simulink model "ZeroForceDrag_SingleJoint"  (R2018b)
settings: Solver=FixedStepDiscrete  StartTime=0.0  StopTime=Inf  FixedStep=0.001  RelTol=1e-3  EnableMultiTasking=on
undefined symbols (not defined in the file): J1, J2, J3, J4, J5, J6, J7, Motor_Current, Motor_Position, Motor_Velocity, Send_GUIdata
libraries: c280xlib x14, simulink x5, idelinklib_common x1
(part 3 of 4)

== system ZeroForceDrag_SingleJoint/DynamicCalculation/GetAngleVelocity/GetAngle2/Joint5 ==
  Action Port : ActionPort  ActionType=case
  Data Store Read5 : DataStoreRead  DataStoreName=Motor_Position  DataStoreElements=Motor_Position(5)
  Joint5 : Outport
  wires:
  Data Store Read5/1 -> Joint5/1

== system ZeroForceDrag_SingleJoint/DynamicCalculation/GetAngleVelocity/GetAngle2/Joint6 ==
  Action Port : ActionPort  ActionType=case
  Data Store Read5 : DataStoreRead  DataStoreName=Motor_Position  DataStoreElements=Motor_Position(6)
  Joint6 : Outport
  wires:
  Data Store Read5/1 -> Joint6/1

== system ZeroForceDrag_SingleJoint/DynamicCalculation/GetAngleVelocity/GetAngle3/Joint1 ==
  note: 内转子位置的脉冲值
  Action Port : ActionPort  ActionType=case
  Data Store Read5 : DataStoreRead  DataStoreName=Motor_Position  DataStoreElements=Motor_Position(1)
  Joint1 : Outport
  wires:
  Data Store Read5/1 -> Joint1/1

== system ZeroForceDrag_SingleJoint/DynamicCalculation/GetAngleVelocity/GetAngle3/Joint2 ==
  Action Port : ActionPort  ActionType=case
  Data Store Read5 : DataStoreRead  DataStoreName=Motor_Position  DataStoreElements=Motor_Position(2)
  Joint2 : Outport
  wires:
  Data Store Read5/1 -> Joint2/1

== system ZeroForceDrag_SingleJoint/DynamicCalculation/GetAngleVelocity/GetAngle3/Joint3 ==
  Action Port : ActionPort  ActionType=case
  Data Store Read5 : DataStoreRead  DataStoreName=Motor_Position  DataStoreElements=Motor_Position(3)
  Joint3 : Outport
  wires:
  Data Store Read5/1 -> Joint3/1

== system ZeroForceDrag_SingleJoint/DynamicCalculation/GetAngleVelocity/GetAngle3/Joint4 ==
  Action Port : ActionPort  ActionType=case
  Data Store Read5 : DataStoreRead  DataStoreName=Motor_Position  DataStoreElements=Motor_Position(4)
  Joint4 : Outport
  wires:
  Data Store Read5/1 -> Joint4/1

== system ZeroForceDrag_SingleJoint/DynamicCalculation/GetAngleVelocity/GetAngle3/Joint5 ==
  Action Port : ActionPort  ActionType=case
  Data Store Read5 : DataStoreRead  DataStoreName=Motor_Position  DataStoreElements=Motor_Position(5)
  Joint5 : Outport
  wires:
  Data Store Read5/1 -> Joint5/1

== system ZeroForceDrag_SingleJoint/DynamicCalculation/GetAngleVelocity/GetAngle3/Joint6 ==
  Action Port : ActionPort  ActionType=case
  Data Store Read5 : DataStoreRead  DataStoreName=Motor_Position  DataStoreElements=Motor_Position(6)
  Joint6 : Outport
  wires:
  Data Store Read5/1 -> Joint6/1

== system ZeroForceDrag_SingleJoint/DynamicCalculation/GetAngleVelocity/GetAngle4/Joint1 ==
  note: 内转子位置的脉冲值
  Action Port : ActionPort  ActionType=case
  Data Store Read5 : DataStoreRead  DataStoreName=Motor_Position  DataStoreElements=Motor_Position(1)
  Joint1 : Outport
  wires:
  Data Store Read5/1 -> Joint1/1

== system ZeroForceDrag_SingleJoint/DynamicCalculation/GetAngleVelocity/GetAngle4/Joint2 ==
  Action Port : ActionPort  ActionType=case
  Data Store Read5 : DataStoreRead  DataStoreName=Motor_Position  DataStoreElements=Motor_Position(2)
  Joint2 : Outport
  wires:
  Data Store Read5/1 -> Joint2/1

== system ZeroForceDrag_SingleJoint/DynamicCalculation/GetAngleVelocity/GetAngle4/Joint3 ==
  Action Port : ActionPort  ActionType=case
  Data Store Read5 : DataStoreRead  DataStoreName=Motor_Position  DataStoreElements=Motor_Position(3)
  Joint3 : Outport
  wires:
  Data Store Read5/1 -> Joint3/1

== system ZeroForceDrag_SingleJoint/DynamicCalculation/GetAngleVelocity/GetAngle4/Joint4 ==
  Action Port : ActionPort  ActionType=case
  Data Store Read5 : DataStoreRead  DataStoreName=Motor_Position  DataStoreElements=Motor_Position(4)
  Joint4 : Outport
  wires:
  Data Store Read5/1 -> Joint4/1

== system ZeroForceDrag_SingleJoint/DynamicCalculation/GetAngleVelocity/GetAngle4/Joint5 ==
  Action Port : ActionPort  ActionType=case
  Data Store Read5 : DataStoreRead  DataStoreName=Motor_Position  DataStoreElements=Motor_Position(5)
  Joint5 : Outport
  wires:
  Data Store Read5/1 -> Joint5/1

== system ZeroForceDrag_SingleJoint/DynamicCalculation/GetAngleVelocity/GetAngle4/Joint6 ==
  Action Port : ActionPort  ActionType=case
  Data Store Read5 : DataStoreRead  DataStoreName=Motor_Position  DataStoreElements=Motor_Position(6)
  Joint6 : Outport
  wires:
  Data Store Read5/1 -> Joint6/1

== system ZeroForceDrag_SingleJoint/DynamicCalculation/GetAngleVelocity/GetAngle5/Joint1 ==
  note: 内转子位置的脉冲值
  Action Port : ActionPort  ActionType=case
  Data Store Read5 : DataStoreRead  DataStoreName=Motor_Position  DataStoreElements=Motor_Position(1)
  Joint1 : Outport
  wires:
  Data Store Read5/1 -> Joint1/1

== system ZeroForceDrag_SingleJoint/DynamicCalculation/GetAngleVelocity/GetAngle5/Joint2 ==
  Action Port : ActionPort  ActionType=case
  Data Store Read5 : DataStoreRead  DataStoreName=Motor_Position  DataStoreElements=Motor_Position(2)
  Joint2 : Outport
  wires:
  Data Store Read5/1 -> Joint2/1

== system ZeroForceDrag_SingleJoint/DynamicCalculation/GetAngleVelocity/GetAngle5/Joint3 ==
  Action Port : ActionPort  ActionType=case
  Data Store Read5 : DataStoreRead  DataStoreName=Motor_Position  DataStoreElements=Motor_Position(3)
  Joint3 : Outport
  wires:
  Data Store Read5/1 -> Joint3/1

== system ZeroForceDrag_SingleJoint/DynamicCalculation/GetAngleVelocity/GetAngle5/Joint4 ==
  Action Port : ActionPort  ActionType=case
  Data Store Read5 : DataStoreRead  DataStoreName=Motor_Position  DataStoreElements=Motor_Position(4)
  Joint4 : Outport
  wires:
  Data Store Read5/1 -> Joint4/1

== system ZeroForceDrag_SingleJoint/DynamicCalculation/GetAngleVelocity/GetAngle5/Joint5 ==
  Action Port : ActionPort  ActionType=case
  Data Store Read5 : DataStoreRead  DataStoreName=Motor_Position  DataStoreElements=Motor_Position(5)
  Joint5 : Outport
  wires:
  Data Store Read5/1 -> Joint5/1

== system ZeroForceDrag_SingleJoint/DynamicCalculation/GetAngleVelocity/GetAngle5/Joint6 ==
  Action Port : ActionPort  ActionType=case
  Data Store Read5 : DataStoreRead  DataStoreName=Motor_Position  DataStoreElements=Motor_Position(6)
  Joint6 : Outport
  wires:
  Data Store Read5/1 -> Joint6/1

== system ZeroForceDrag_SingleJoint/DynamicCalculation/GetAngleVelocity/GetAngle6/Joint1 ==
  note: 内转子位置的脉冲值
  Action Port : ActionPort  ActionType=case
  Data Store Read5 : DataStoreRead  DataStoreName=Motor_Position  DataStoreElements=Motor_Position(1)
  Joint1 : Outport
  wires:
  Data Store Read5/1 -> Joint1/1

== system ZeroForceDrag_SingleJoint/DynamicCalculation/GetAngleVelocity/GetAngle6/Joint2 ==
  Action Port : ActionPort  ActionType=case
  Data Store Read5 : DataStoreRead  DataStoreName=Motor_Position  DataStoreElements=Motor_Position(2)
  Joint2 : Outport
  wires:
  Data Store Read5/1 -> Joint2/1

== system ZeroForceDrag_SingleJoint/DynamicCalculation/GetAngleVelocity/GetAngle6/Joint3 ==
  Action Port : ActionPort  ActionType=case
  Data Store Read5 : DataStoreRead  DataStoreName=Motor_Position  DataStoreElements=Motor_Position(3)
  Joint3 : Outport
  wires:
  Data Store Read5/1 -> Joint3/1

== system ZeroForceDrag_SingleJoint/DynamicCalculation/GetAngleVelocity/GetAngle6/Joint4 ==
  Action Port : ActionPort  ActionType=case
  Data Store Read5 : DataStoreRead  DataStoreName=Motor_Position  DataStoreElements=Motor_Position(4)
  Joint4 : Outport
  wires:
  Data Store Read5/1 -> Joint4/1

== system ZeroForceDrag_SingleJoint/DynamicCalculation/GetAngleVelocity/GetAngle6/Joint5 ==
  Action Port : ActionPort  ActionType=case
  Data Store Read5 : DataStoreRead  DataStoreName=Motor_Position  DataStoreElements=Motor_Position(5)
  Joint5 : Outport
  wires:
  Data Store Read5/1 -> Joint5/1

== system ZeroForceDrag_SingleJoint/DynamicCalculation/GetAngleVelocity/GetAngle6/Joint6 ==
  Action Port : ActionPort  ActionType=case
  Data Store Read5 : DataStoreRead  DataStoreName=Motor_Position  DataStoreElements=Motor_Position(6)
  Joint6 : Outport
  wires:
  Data Store Read5/1 -> Joint6/1

== system ZeroForceDrag_SingleJoint/DynamicCalculation/GetAngleVelocity/GetAngleSpeed/Joint1 ==
  note: 内转子速度
      | 的脉冲值
  Action Port : ActionPort  ActionType=case
  Data Store Read1 : DataStoreRead  DataStoreName=Motor_Velocity  DataStoreElements=Motor_Velocity(1)
  Joint1_Velocity : Outport
  wires:
  Data Store Read1/1 -> Joint1_Velocity/1

== system ZeroForceDrag_SingleJoint/DynamicCalculation/GetAngleVelocity/GetAngleSpeed/Joint2 ==
  note: 内转子速度
      | 的脉冲值
  Action Port : ActionPort  ActionType=case
  Data Store Read1 : DataStoreRead  DataStoreName=Motor_Velocity  DataStoreElements=Motor_Velocity(2)
  Joint2_Velocity : Outport
  wires:
  Data Store Read1/1 -> Joint2_Velocity/1

== system ZeroForceDrag_SingleJoint/DynamicCalculation/GetAngleVelocity/GetAngleSpeed/Joint3 ==
  note: 内转子速度
      | 的脉冲值
  Action Port : ActionPort  ActionType=case
  Data Store Read1 : DataStoreRead  DataStoreName=Motor_Velocity  DataStoreElements=Motor_Velocity(3)
  Joint3_Velocity : Outport
  wires:
  Data Store Read1/1 -> Joint3_Velocity/1

== system ZeroForceDrag_SingleJoint/DynamicCalculation/GetAngleVelocity/GetAngleSpeed/Joint4 ==
  note: 内转子速度
      | 的脉冲值
  Action Port : ActionPort  ActionType=case
  Data Store Read1 : DataStoreRead  DataStoreName=Motor_Velocity  DataStoreElements=Motor_Velocity(4)
  Joint4_Velocity : Outport
  wires:
  Data Store Read1/1 -> Joint4_Velocity/1

== system ZeroForceDrag_SingleJoint/DynamicCalculation/GetAngleVelocity/GetAngleSpeed/Joint5 ==
  note: 内转子速度
      | 的脉冲值
  Action Port : ActionPort  ActionType=case
  Data Store Read1 : DataStoreRead  DataStoreName=Motor_Velocity  DataStoreElements=Motor_Velocity(5)
  Joint5_Velocity : Outport
  wires:
  Data Store Read1/1 -> Joint5_Velocity/1

== system ZeroForceDrag_SingleJoint/DynamicCalculation/GetAngleVelocity/GetAngleSpeed/Joint6 ==
  note: 内转子速度
      | 的脉冲值
  Action Port : ActionPort  ActionType=case
  Data Store Read1 : DataStoreRead  DataStoreName=Motor_Velocity  DataStoreElements=Motor_Velocity(6)
  Joint6_Velocity : Outport
  wires:
  Data Store Read1/1 -> Joint6_Velocity/1

== system ZeroForceDrag_SingleJoint/DynamicCalculation/GetAngleVelocity/GetAngleSpeed1/Joint1 ==
  note: 内转子速度
      | 的脉冲值
  Action Port : ActionPort  ActionType=case
  Data Store Read1 : DataStoreRead  DataStoreName=Motor_Velocity  DataStoreElements=Motor_Velocity(1)
  Joint1_Velocity : Outport
  wires:
  Data Store Read1/1 -> Joint1_Velocity/1

== system ZeroForceDrag_SingleJoint/DynamicCalculation/GetAngleVelocity/GetAngleSpeed1/Joint2 ==
  note: 内转子速度
      | 的脉冲值
  Action Port : ActionPort  ActionType=case
  Data Store Read1 : DataStoreRead  DataStoreName=Motor_Velocity  DataStoreElements=Motor_Velocity(2)
  Joint2_Velocity : Outport
  wires:
  Data Store Read1/1 -> Joint2_Velocity/1

== system ZeroForceDrag_SingleJoint/DynamicCalculation/GetAngleVelocity/GetAngleSpeed1/Joint3 ==
  note: 内转子速度
      | 的脉冲值
  Action Port : ActionPort  ActionType=case
  Data Store Read1 : DataStoreRead  DataStoreName=Motor_Velocity  DataStoreElements=Motor_Velocity(3)
  Joint3_Velocity : Outport
  wires:
  Data Store Read1/1 -> Joint3_Velocity/1

== system ZeroForceDrag_SingleJoint/DynamicCalculation/GetAngleVelocity/GetAngleSpeed1/Joint4 ==
  note: 内转子速度
      | 的脉冲值
  Action Port : ActionPort  ActionType=case
  Data Store Read1 : DataStoreRead  DataStoreName=Motor_Velocity  DataStoreElements=Motor_Velocity(4)
  Joint4_Velocity : Outport
  wires:
  Data Store Read1/1 -> Joint4_Velocity/1

== system ZeroForceDrag_SingleJoint/DynamicCalculation/GetAngleVelocity/GetAngleSpeed1/Joint5 ==
  note: 内转子速度
      | 的脉冲值
  Action Port : ActionPort  ActionType=case
  Data Store Read1 : DataStoreRead  DataStoreName=Motor_Velocity  DataStoreElements=Motor_Velocity(5)
  Joint5_Velocity : Outport
  wires:
  Data Store Read1/1 -> Joint5_Velocity/1

== system ZeroForceDrag_SingleJoint/DynamicCalculation/GetAngleVelocity/GetAngleSpeed1/Joint6 ==
  note: 内转子速度
      | 的脉冲值
  Action Port : ActionPort  ActionType=case
  Data Store Read1 : DataStoreRead  DataStoreName=Motor_Velocity  DataStoreElements=Motor_Velocity(6)
  Joint6_Velocity : Outport
  wires:
  Data Store Read1/1 -> Joint6_Velocity/1

== system ZeroForceDrag_SingleJoint/DynamicCalculation/GetAngleVelocity/GetAngleSpeed2/Joint1 ==
  note: 内转子速度
      | 的脉冲值
  Action Port : ActionPort  ActionType=case
  Data Store Read1 : DataStoreRead  DataStoreName=Motor_Velocity  DataStoreElements=Motor_Velocity(1)
  Joint1_Velocity : Outport
  wires:
  Data Store Read1/1 -> Joint1_Velocity/1

== system ZeroForceDrag_SingleJoint/DynamicCalculation/GetAngleVelocity/GetAngleSpeed2/Joint2 ==
  note: 内转子速度
      | 的脉冲值
  Action Port : ActionPort  ActionType=case
  Data Store Read1 : DataStoreRead  DataStoreName=Motor_Velocity  DataStoreElements=Motor_Velocity(2)
  Joint2_Velocity : Outport
  wires:
  Data Store Read1/1 -> Joint2_Velocity/1

== system ZeroForceDrag_SingleJoint/DynamicCalculation/GetAngleVelocity/GetAngleSpeed2/Joint3 ==
  note: 内转子速度
      | 的脉冲值
  Action Port : ActionPort  ActionType=case
  Data Store Read1 : DataStoreRead  DataStoreName=Motor_Velocity  DataStoreElements=Motor_Velocity(3)
  Joint3_Velocity : Outport
  wires:
  Data Store Read1/1 -> Joint3_Velocity/1

== system ZeroForceDrag_SingleJoint/DynamicCalculation/GetAngleVelocity/GetAngleSpeed2/Joint4 ==
  note: 内转子速度
      | 的脉冲值
  Action Port : ActionPort  ActionType=case
  Data Store Read1 : DataStoreRead  DataStoreName=Motor_Velocity  DataStoreElements=Motor_Velocity(4)
  Joint4_Velocity : Outport
  wires:
  Data Store Read1/1 -> Joint4_Velocity/1

== system ZeroForceDrag_SingleJoint/DynamicCalculation/GetAngleVelocity/GetAngleSpeed2/Joint5 ==
  note: 内转子速度
      | 的脉冲值
  Action Port : ActionPort  ActionType=case
  Data Store Read1 : DataStoreRead  DataStoreName=Motor_Velocity  DataStoreElements=Motor_Velocity(5)
  Joint5_Velocity : Outport
  wires:
  Data Store Read1/1 -> Joint5_Velocity/1

== system ZeroForceDrag_SingleJoint/DynamicCalculation/GetAngleVelocity/GetAngleSpeed2/Joint6 ==
  note: 内转子速度
      | 的脉冲值
  Action Port : ActionPort  ActionType=case
  Data Store Read1 : DataStoreRead  DataStoreName=Motor_Velocity  DataStoreElements=Motor_Velocity(6)
  Joint6_Velocity : Outport
  wires:
  Data Store Read1/1 -> Joint6_Velocity/1

== system ZeroForceDrag_SingleJoint/DynamicCalculation/GetAngleVelocity/GetAngleSpeed3/Joint1 ==
  note: 内转子速度
      | 的脉冲值
  Action Port : ActionPort  ActionType=case
  Data Store Read1 : DataStoreRead  DataStoreName=Motor_Velocity  DataStoreElements=Motor_Velocity(1)
  Joint1_Velocity : Outport
  wires:
  Data Store Read1/1 -> Joint1_Velocity/1

== system ZeroForceDrag_SingleJoint/DynamicCalculation/GetAngleVelocity/GetAngleSpeed3/Joint2 ==
  note: 内转子速度
      | 的脉冲值
  Action Port : ActionPort  ActionType=case
  Data Store Read1 : DataStoreRead  DataStoreName=Motor_Velocity  DataStoreElements=Motor_Velocity(2)
  Joint2_Velocity : Outport
  wires:
  Data Store Read1/1 -> Joint2_Velocity/1

== system ZeroForceDrag_SingleJoint/DynamicCalculation/GetAngleVelocity/GetAngleSpeed3/Joint3 ==
  note: 内转子速度
      | 的脉冲值
  Action Port : ActionPort  ActionType=case
  Data Store Read1 : DataStoreRead  DataStoreName=Motor_Velocity  DataStoreElements=Motor_Velocity(3)
  Joint3_Velocity : Outport
  wires:
  Data Store Read1/1 -> Joint3_Velocity/1

== system ZeroForceDrag_SingleJoint/DynamicCalculation/GetAngleVelocity/GetAngleSpeed3/Joint4 ==
  note: 内转子速度
      | 的脉冲值
  Action Port : ActionPort  ActionType=case
  Data Store Read1 : DataStoreRead  DataStoreName=Motor_Velocity  DataStoreElements=Motor_Velocity(4)
  Joint4_Velocity : Outport
  wires:
  Data Store Read1/1 -> Joint4_Velocity/1

== system ZeroForceDrag_SingleJoint/DynamicCalculation/GetAngleVelocity/GetAngleSpeed3/Joint5 ==
  note: 内转子速度
      | 的脉冲值
  Action Port : ActionPort  ActionType=case
  Data Store Read1 : DataStoreRead  DataStoreName=Motor_Velocity  DataStoreElements=Motor_Velocity(5)
  Joint5_Velocity : Outport
  wires:
  Data Store Read1/1 -> Joint5_Velocity/1

== system ZeroForceDrag_SingleJoint/DynamicCalculation/GetAngleVelocity/GetAngleSpeed3/Joint6 ==
  note: 内转子速度
      | 的脉冲值
  Action Port : ActionPort  ActionType=case
  Data Store Read1 : DataStoreRead  DataStoreName=Motor_Velocity  DataStoreElements=Motor_Velocity(6)
  Joint6_Velocity : Outport
  wires:
  Data Store Read1/1 -> Joint6_Velocity/1

== system ZeroForceDrag_SingleJoint/DynamicCalculation/GetAngleVelocity/GetAngleSpeed4/Joint1 ==
  note: 内转子速度
      | 的脉冲值
  Action Port : ActionPort  ActionType=case
  Data Store Read1 : DataStoreRead  DataStoreName=Motor_Velocity  DataStoreElements=Motor_Velocity(1)
  Joint1_Velocity : Outport
  wires:
  Data Store Read1/1 -> Joint1_Velocity/1

== system ZeroForceDrag_SingleJoint/DynamicCalculation/GetAngleVelocity/GetAngleSpeed4/Joint2 ==
  note: 内转子速度
      | 的脉冲值
  Action Port : ActionPort  ActionType=case
  Data Store Read1 : DataStoreRead  DataStoreName=Motor_Velocity  DataStoreElements=Motor_Velocity(2)
  Joint2_Velocity : Outport
  wires:
  Data Store Read1/1 -> Joint2_Velocity/1

== system ZeroForceDrag_SingleJoint/DynamicCalculation/GetAngleVelocity/GetAngleSpeed4/Joint3 ==
  note: 内转子速度
      | 的脉冲值
  Action Port : ActionPort  ActionType=case
  Data Store Read1 : DataStoreRead  DataStoreName=Motor_Velocity  DataStoreElements=Motor_Velocity(3)
  Joint3_Velocity : Outport
  wires:
  Data Store Read1/1 -> Joint3_Velocity/1

== system ZeroForceDrag_SingleJoint/DynamicCalculation/GetAngleVelocity/GetAngleSpeed4/Joint4 ==
  note: 内转子速度
      | 的脉冲值
  Action Port : ActionPort  ActionType=case
  Data Store Read1 : DataStoreRead  DataStoreName=Motor_Velocity  DataStoreElements=Motor_Velocity(4)
  Joint4_Velocity : Outport
  wires:
  Data Store Read1/1 -> Joint4_Velocity/1

== system ZeroForceDrag_SingleJoint/DynamicCalculation/GetAngleVelocity/GetAngleSpeed4/Joint5 ==
  note: 内转子速度
      | 的脉冲值
  Action Port : ActionPort  ActionType=case
  Data Store Read1 : DataStoreRead  DataStoreName=Motor_Velocity  DataStoreElements=Motor_Velocity(5)
  Joint5_Velocity : Outport
  wires:
  Data Store Read1/1 -> Joint5_Velocity/1

== system ZeroForceDrag_SingleJoint/DynamicCalculation/GetAngleVelocity/GetAngleSpeed4/Joint6 ==
  note: 内转子速度
      | 的脉冲值
  Action Port : ActionPort  ActionType=case
  Data Store Read1 : DataStoreRead  DataStoreName=Motor_Velocity  DataStoreElements=Motor_Velocity(6)
  Joint6_Velocity : Outport
  wires:
  Data Store Read1/1 -> Joint6_Velocity/1

== system ZeroForceDrag_SingleJoint/DynamicCalculation/GetAngleVelocity/GetAngleSpeed5/Joint1 ==
  note: 内转子速度
      | 的脉冲值
  Action Port : ActionPort  ActionType=case
  Data Store Read1 : DataStoreRead  DataStoreName=Motor_Velocity  DataStoreElements=Motor_Velocity(1)
  Joint1_Velocity : Outport
  wires:
  Data Store Read1/1 -> Joint1_Velocity/1

== system ZeroForceDrag_SingleJoint/DynamicCalculation/GetAngleVelocity/GetAngleSpeed5/Joint2 ==
  note: 内转子速度
      | 的脉冲值
  Action Port : ActionPort  ActionType=case
  Data Store Read1 : DataStoreRead  DataStoreName=Motor_Velocity  DataStoreElements=Motor_Velocity(2)
  Joint2_Velocity : Outport
  wires:
  Data Store Read1/1 -> Joint2_Velocity/1

== system ZeroForceDrag_SingleJoint/DynamicCalculation/GetAngleVelocity/GetAngleSpeed5/Joint3 ==
  note: 内转子速度
      | 的脉冲值
  Action Port : ActionPort  ActionType=case
  Data Store Read1 : DataStoreRead  DataStoreName=Motor_Velocity  DataStoreElements=Motor_Velocity(3)
  Joint3_Velocity : Outport
  wires:
  Data Store Read1/1 -> Joint3_Velocity/1

== system ZeroForceDrag_SingleJoint/DynamicCalculation/GetAngleVelocity/GetAngleSpeed5/Joint4 ==
  note: 内转子速度
      | 的脉冲值
  Action Port : ActionPort  ActionType=case
  Data Store Read1 : DataStoreRead  DataStoreName=Motor_Velocity  DataStoreElements=Motor_Velocity(4)
  Joint4_Velocity : Outport
  wires:
  Data Store Read1/1 -> Joint4_Velocity/1

== system ZeroForceDrag_SingleJoint/DynamicCalculation/GetAngleVelocity/GetAngleSpeed5/Joint5 ==
  note: 内转子速度
      | 的脉冲值
  Action Port : ActionPort  ActionType=case
  Data Store Read1 : DataStoreRead  DataStoreName=Motor_Velocity  DataStoreElements=Motor_Velocity(5)
  Joint5_Velocity : Outport
  wires:
  Data Store Read1/1 -> Joint5_Velocity/1

== system ZeroForceDrag_SingleJoint/DynamicCalculation/GetAngleVelocity/GetAngleSpeed5/Joint6 ==
  note: 内转子速度
      | 的脉冲值
  Action Port : ActionPort  ActionType=case
  Data Store Read1 : DataStoreRead  DataStoreName=Motor_Velocity  DataStoreElements=Motor_Velocity(6)
  Joint6_Velocity : Outport
  wires:
  Data Store Read1/1 -> Joint6_Velocity/1

== system ZeroForceDrag_SingleJoint/DynamicCalculation/DriveMotor/驱动器指令/Chart2/BG/J1_BG ==
  note: 命令
  note: 电流
  note: 位
      | 置
  Constant1 : Constant  Value=hex2dec('47')  OutDataTypeStr=uint8
  Constant2 : Constant  Value=0  VectorParams1D=off  OutDataTypeStr=uint8  SampleTime=-1
  Constant3 : Constant  Value=0  VectorParams1D=off  OutDataTypeStr=uint8  SampleTime=-1
  Constant8 : Constant  Value=hex2dec('42')  OutDataTypeStr=uint8
  Data Type Conversion : DataTypeConversion  OutDataTypeStr=uint16
  Data Type Conversion{1..6} (6 alike) : DataTypeConversion  OutDataTypeStr=uint8
  Mux3 : Mux  Inputs=8
  Shift Arithmetic1 : ArithShift  BitShiftNumber=8  BitShiftDirection=Right
  Shift Arithmetic2 : ArithShift  BitShiftNumber=16  BitShiftDirection=Right
  Shift Arithmetic3 : ArithShift  BitShiftNumber=24  BitShiftDirection=Right
  Shift Arithmetic4 : ArithShift  BitShiftNumber=8  BitShiftDirection=Right
  MSG : Outport
  wires:
  Shift Arithmetic2/1 -> Data Type Conversion4/1
  Shift Arithmetic4/1 -> Data Type Conversion6/1
  Constant2/1 -> Shift Arithmetic4/1, Data Type Conversion1/1
  Data Type Conversion1/1 -> Mux3/3
  Data Type Conversion3/1 -> Mux3/6
  Constant3/1 -> Data Type Conversion2/1, Shift Arithmetic1/1, Shift Arithmetic2/1, Shift Arithmetic3/1
  Data Type Conversion6/1 -> Mux3/4
  Shift Arithmetic3/1 -> Data Type Conversion5/1
  Shift Arithmetic1/1 -> Data Type Conversion3/1
  Mux3/1 -> Data Type Conversion/1
  Data Type Conversion2/1 -> Mux3/5
  Constant8/1 -> Mux3/1
  Data Type Conversion4/1 -> Mux3/7
  Data Type Conversion5/1 -> Mux3/8
  Constant1/1 -> Mux3/2
  Data Type Conversion/1 -> MSG/1

== system ZeroForceDrag_SingleJoint/DynamicCalculation/DriveMotor/驱动器指令/Chart2/BG/J2_BG ==
  note: 位
      | 置
  note: 电流
  note: 命令
  Constant1 : Constant  Value=hex2dec('47')  OutDataTypeStr=uint8
  Constant2 : Constant  Value=0  VectorParams1D=off  OutDataTypeStr=uint8  SampleTime=-1
  Constant3 : Constant  Value=0  VectorParams1D=off  OutDataTypeStr=uint8  SampleTime=-1
  Constant8 : Constant  Value=hex2dec('42')  OutDataTypeStr=uint8
  Data Type Conversion : DataTypeConversion  OutDataTypeStr=uint16
  Data Type Conversion{1..6} (6 alike) : DataTypeConversion  OutDataTypeStr=uint8
  Mux3 : Mux  Inputs=8
  Shift Arithmetic1 : ArithShift  BitShiftNumber=8  BitShiftDirection=Right
  Shift Arithmetic2 : ArithShift  BitShiftNumber=16  BitShiftDirection=Right
  Shift Arithmetic3 : ArithShift  BitShiftNumber=24  BitShiftDirection=Right
  Shift Arithmetic4 : ArithShift  BitShiftNumber=8  BitShiftDirection=Right
  MSG : Outport
  wires:
  Data Type Conversion/1 -> MSG/1
  Constant1/1 -> Mux3/2
  Data Type Conversion5/1 -> Mux3/8
  Data Type Conversion4/1 -> Mux3/7
  Constant8/1 -> Mux3/1
  Data Type Conversion2/1 -> Mux3/5
  Mux3/1 -> Data Type Conversion/1
  Shift Arithmetic1/1 -> Data Type Conversion3/1
  Shift Arithmetic3/1 -> Data Type Conversion5/1
  Data Type Conversion6/1 -> Mux3/4
  Constant3/1 -> Shift Arithmetic3/1, Shift Arithmetic2/1, Shift Arithmetic1/1, Data Type Conversion2/1
  Data Type Conversion3/1 -> Mux3/6
  Data Type Conversion1/1 -> Mux3/3
  Constant2/1 -> Data Type Conversion1/1, Shift Arithmetic4/1
  Shift Arithmetic4/1 -> Data Type Conversion6/1
  Shift Arithmetic2/1 -> Data Type Conversion4/1

== system ZeroForceDrag_SingleJoint/DynamicCalculation/DriveMotor/驱动器指令/Chart2/BG/J3_BG ==
  note: 命令
  note: 电流
  note: 位
      | 置
  Constant1 : Constant  Value=hex2dec('47')  OutDataTypeStr=uint8
  Constant2 : Constant  Value=0  VectorParams1D=off  OutDataTypeStr=uint8  SampleTime=-1
  Constant3 : Constant  Value=0  VectorParams1D=off  OutDataTypeStr=uint8  SampleTime=-1
  Constant8 : Constant  Value=hex2dec('42')  OutDataTypeStr=uint8
  Data Type Conversion : DataTypeConversion  OutDataTypeStr=uint16
  Data Type Conversion{1..6} (6 alike) : DataTypeConversion  OutDataTypeStr=uint8
  Mux3 : Mux  Inputs=8
  Shift Arithmetic1 : ArithShift  BitShiftNumber=8  BitShiftDirection=Right
  Shift Arithmetic2 : ArithShift  BitShiftNumber=16  BitShiftDirection=Right
  Shift Arithmetic3 : ArithShift  BitShiftNumber=24  BitShiftDirection=Right
  Shift Arithmetic4 : ArithShift  BitShiftNumber=8  BitShiftDirection=Right
  MSG : Outport
  wires:
  Shift Arithmetic2/1 -> Data Type Conversion4/1
  Shift Arithmetic4/1 -> Data Type Conversion6/1
  Constant2/1 -> Shift Arithmetic4/1, Data Type Conversion1/1
  Data Type Conversion1/1 -> Mux3/3
  Data Type Conversion3/1 -> Mux3/6
  Constant3/1 -> Data Type Conversion2/1, Shift Arithmetic1/1, Shift Arithmetic2/1, Shift Arithmetic3/1
  Data Type Conversion6/1 -> Mux3/4
  Shift Arithmetic3/1 -> Data Type Conversion5/1
  Shift Arithmetic1/1 -> Data Type Conversion3/1
  Mux3/1 -> Data Type Conversion/1
  Data Type Conversion2/1 -> Mux3/5
  Constant8/1 -> Mux3/1
  Data Type Conversion4/1 -> Mux3/7
  Data Type Conversion5/1 -> Mux3/8
  Constant1/1 -> Mux3/2
  Data Type Conversion/1 -> MSG/1

== system ZeroForceDrag_SingleJoint/DynamicCalculation/DriveMotor/驱动器指令/Chart2/BG/J4_BG ==
  note: 位
      | 置
  note: 电流
  note: 命令
  Constant1 : Constant  Value=hex2dec('47')  OutDataTypeStr=uint8
  Constant2 : Constant  Value=0  VectorParams1D=off  OutDataTypeStr=uint8  SampleTime=-1
  Constant3 : Constant  Value=0  VectorParams1D=off  OutDataTypeStr=uint8  SampleTime=-1
  Constant8 : Constant  Value=hex2dec('42')  OutDataTypeStr=uint8
  Data Type Conversion : DataTypeConversion  OutDataTypeStr=uint16
  Data Type Conversion{1..6} (6 alike) : DataTypeConversion  OutDataTypeStr=uint8
  Mux3 : Mux  Inputs=8
  Shift Arithmetic1 : ArithShift  BitShiftNumber=8  BitShiftDirection=Right
  Shift Arithmetic2 : ArithShift  BitShiftNumber=16  BitShiftDirection=Right
  Shift Arithmetic3 : ArithShift  BitShiftNumber=24  BitShiftDirection=Right
  Shift Arithmetic4 : ArithShift  BitShiftNumber=8  BitShiftDirection=Right
  MSG : Outport
  wires:
  Data Type Conversion/1 -> MSG/1
  Constant1/1 -> Mux3/2
  Data Type Conversion5/1 -> Mux3/8
  Data Type Conversion4/1 -> Mux3/7
  Constant8/1 -> Mux3/1
  Data Type Conversion2/1 -> Mux3/5
  Mux3/1 -> Data Type Conversion/1
  Shift Arithmetic1/1 -> Data Type Conversion3/1
  Shift Arithmetic3/1 -> Data Type Conversion5/1
  Data Type Conversion6/1 -> Mux3/4
  Constant3/1 -> Shift Arithmetic3/1, Shift Arithmetic2/1, Shift Arithmetic1/1, Data Type Conversion2/1
  Data Type Conversion3/1 -> Mux3/6
  Data Type Conversion1/1 -> Mux3/3
  Constant2/1 -> Data Type Conversion1/1, Shift Arithmetic4/1
  Shift Arithmetic4/1 -> Data Type Conversion6/1
  Shift Arithmetic2/1 -> Data Type Conversion4/1

== system ZeroForceDrag_SingleJoint/DynamicCalculation/DriveMotor/驱动器指令/Chart2/BG/J5_BG ==
  note: 命令
  note: 电流
  note: 位
      | 置
  Constant1 : Constant  Value=hex2dec('47')  OutDataTypeStr=uint8
  Constant2 : Constant  Value=0  VectorParams1D=off  OutDataTypeStr=uint8  SampleTime=-1
  Constant3 : Constant  Value=0  VectorParams1D=off  OutDataTypeStr=uint8  SampleTime=-1
  Constant8 : Constant  Value=hex2dec('42')  OutDataTypeStr=uint8
  Data Type Conversion : DataTypeConversion  OutDataTypeStr=uint16
  Data Type Conversion{1..6} (6 alike) : DataTypeConversion  OutDataTypeStr=uint8
  Mux3 : Mux  Inputs=8
  Shift Arithmetic1 : ArithShift  BitShiftNumber=8  BitShiftDirection=Right
  Shift Arithmetic2 : ArithShift  BitShiftNumber=16  BitShiftDirection=Right
  Shift Arithmetic3 : ArithShift  BitShiftNumber=24  BitShiftDirection=Right
  Shift Arithmetic4 : ArithShift  BitShiftNumber=8  BitShiftDirection=Right
  MSG : Outport
  wires:
  Shift Arithmetic2/1 -> Data Type Conversion4/1
  Shift Arithmetic4/1 -> Data Type Conversion6/1
  Constant2/1 -> Shift Arithmetic4/1, Data Type Conversion1/1
  Data Type Conversion1/1 -> Mux3/3
  Data Type Conversion3/1 -> Mux3/6
  Constant3/1 -> Data Type Conversion2/1, Shift Arithmetic1/1, Shift Arithmetic2/1, Shift Arithmetic3/1
  Data Type Conversion6/1 -> Mux3/4
  Shift Arithmetic3/1 -> Data Type Conversion5/1
  Shift Arithmetic1/1 -> Data Type Conversion3/1
  Mux3/1 -> Data Type Conversion/1
  Data Type Conversion2/1 -> Mux3/5
  Constant8/1 -> Mux3/1
  Data Type Conversion4/1 -> Mux3/7
  Data Type Conversion5/1 -> Mux3/8
  Constant1/1 -> Mux3/2
  Data Type Conversion/1 -> MSG/1

== system ZeroForceDrag_SingleJoint/DynamicCalculation/DriveMotor/驱动器指令/Chart2/BG/J6_BG ==
  note: 位
      | 置
  note: 电流
  note: 命令
  Constant1 : Constant  Value=hex2dec('47')  OutDataTypeStr=uint8
  Constant2 : Constant  Value=0  VectorParams1D=off  OutDataTypeStr=uint8  SampleTime=-1
  Constant3 : Constant  Value=0  VectorParams1D=off  OutDataTypeStr=uint8  SampleTime=-1
  Constant8 : Constant  Value=hex2dec('42')  OutDataTypeStr=uint8
  Data Type Conversion : DataTypeConversion  OutDataTypeStr=uint16
  Data Type Conversion{1..6} (6 alike) : DataTypeConversion  OutDataTypeStr=uint8
  Mux3 : Mux  Inputs=8
  Shift Arithmetic1 : ArithShift  BitShiftNumber=8  BitShiftDirection=Right
  Shift Arithmetic2 : ArithShift  BitShiftNumber=16  BitShiftDirection=Right
  Shift Arithmetic3 : ArithShift  BitShiftNumber=24  BitShiftDirection=Right
  Shift Arithmetic4 : ArithShift  BitShiftNumber=8  BitShiftDirection=Right
  MSG : Outport
  wires:
  Data Type Conversion/1 -> MSG/1
  Constant1/1 -> Mux3/2
  Data Type Conversion5/1 -> Mux3/8
  Data Type Conversion4/1 -> Mux3/7
  Constant8/1 -> Mux3/1
  Data Type Conversion2/1 -> Mux3/5
  Mux3/1 -> Data Type Conversion/1
  Shift Arithmetic1/1 -> Data Type Conversion3/1
  Shift Arithmetic3/1 -> Data Type Conversion5/1
  Data Type Conversion6/1 -> Mux3/4
  Constant3/1 -> Shift Arithmetic3/1, Shift Arithmetic2/1, Shift Arithmetic1/1, Data Type Conversion2/1
  Data Type Conversion3/1 -> Mux3/6
  Data Type Conversion1/1 -> Mux3/3
  Constant2/1 -> Data Type Conversion1/1, Shift Arithmetic4/1
  Shift Arithmetic4/1 -> Data Type Conversion6/1
  Shift Arithmetic2/1 -> Data Type Conversion4/1

== system ZeroForceDrag_SingleJoint/DynamicCalculation/DriveMotor/驱动器指令/Chart2/TF/J1_TF ==
  note: 命令
  note: 位
      | 置
  note: 电流
  Current : Inport
  Constant1 : Constant  Value=hex2dec('46')  OutDataTypeStr=uint8
  Constant3 : Constant  Value=0  VectorParams1D=off  OutDataTypeStr=uint8  SampleTime=-1
  Constant8 : Constant  Value=hex2dec('54')  OutDataTypeStr=uint8
  Data Type Conversion : DataTypeConversion  OutDataTypeStr=uint16
  Data Type Conversion{1..6} (6 alike) : DataTypeConversion  OutDataTypeStr=uint8
  Mux3 : Mux  Inputs=8
  Shift Arithmetic1 : ArithShift  BitShiftNumber=8  BitShiftDirection=Right
  Shift Arithmetic2 : ArithShift  BitShiftNumber=16  BitShiftDirection=Right
  Shift Arithmetic3 : ArithShift  BitShiftNumber=24  BitShiftDirection=Right
  Shift Arithmetic4 : ArithShift  BitShiftNumber=8  BitShiftDirection=Right
  MSG : Outport  OutDataTypeStr=uint16
  wires:
  Shift Arithmetic1/1 -> Data Type Conversion3/1
  Shift Arithmetic3/1 -> Data Type Conversion5/1
  Constant3/1 -> Shift Arithmetic3/1, Shift Arithmetic2/1, Shift Arithmetic1/1, Data Type Conversion2/1
  Mux3/1 -> Data Type Conversion/1
  Constant8/1 -> Mux3/1
  Data Type Conversion3/1 -> Mux3/6
  Data Type Conversion2/1 -> Mux3/5
  Data Type Conversion1/1 -> Mux3/3
  Data Type Conversion5/1 -> Mux3/8
  Current/1 -> Shift Arithmetic4/1, Data Type Conversion1/1
  Shift Arithmetic2/1 -> Data Type Conversion4/1
  Constant1/1 -> Mux3/2
  Data Type Conversion6/1 -> Mux3/4
  Shift Arithmetic4/1 -> Data Type Conversion6/1
  Data Type Conversion4/1 -> Mux3/7
  Data Type Conversion/1 -> MSG/1

== system ZeroForceDrag_SingleJoint/DynamicCalculation/DriveMotor/驱动器指令/Chart2/TF/J2_TF ==
  note: 电流
  note: 位
      | 置
  note: 命令
  Current : Inport
  Constant1 : Constant  Value=hex2dec('46')  OutDataTypeStr=uint8
  Constant3 : Constant  Value=0  VectorParams1D=off  OutDataTypeStr=uint8  SampleTime=-1
  Constant8 : Constant  Value=hex2dec('54')  OutDataTypeStr=uint8
  Data Type Conversion : DataTypeConversion  OutDataTypeStr=uint16
  Data Type Conversion{1..6} (6 alike) : DataTypeConversion  OutDataTypeStr=uint8
  Mux3 : Mux  Inputs=8
  Shift Arithmetic1 : ArithShift  BitShiftNumber=8  BitShiftDirection=Right
  Shift Arithmetic2 : ArithShift  BitShiftNumber=16  BitShiftDirection=Right
  Shift Arithmetic3 : ArithShift  BitShiftNumber=24  BitShiftDirection=Right
  Shift Arithmetic4 : ArithShift  BitShiftNumber=8  BitShiftDirection=Right
  MSG : Outport  OutDataTypeStr=uint16
  wires:
  Data Type Conversion/1 -> MSG/1
  Data Type Conversion4/1 -> Mux3/7
  Shift Arithmetic4/1 -> Data Type Conversion6/1
  Data Type Conversion6/1 -> Mux3/4
  Constant1/1 -> Mux3/2
  Shift Arithmetic2/1 -> Data Type Conversion4/1
  Current/1 -> Data Type Conversion1/1, Shift Arithmetic4/1
  Data Type Conversion5/1 -> Mux3/8
  Data Type Conversion1/1 -> Mux3/3
  Data Type Conversion2/1 -> Mux3/5
  Data Type Conversion3/1 -> Mux3/6
  Constant8/1 -> Mux3/1
  Mux3/1 -> Data Type Conversion/1
  Constant3/1 -> Data Type Conversion2/1, Shift Arithmetic1/1, Shift Arithmetic2/1, Shift Arithmetic3/1
  Shift Arithmetic3/1 -> Data Type Conversion5/1
  Shift Arithmetic1/1 -> Data Type Conversion3/1

== system ZeroForceDrag_SingleJoint/DynamicCalculation/DriveMotor/驱动器指令/Chart2/TF/J3_TF ==
  note: 命令
  note: 位
      | 置
  note: 电流
  Current : Inport
  Constant1 : Constant  Value=hex2dec('46')  OutDataTypeStr=uint8
  Constant3 : Constant  Value=0  VectorParams1D=off  OutDataTypeStr=uint8  SampleTime=-1
  Constant8 : Constant  Value=hex2dec('54')  OutDataTypeStr=uint8
  Data Type Conversion : DataTypeConversion  OutDataTypeStr=uint16
  Data Type Conversion{1..6} (6 alike) : DataTypeConversion  OutDataTypeStr=uint8
  Mux3 : Mux  Inputs=8
  Shift Arithmetic1 : ArithShift  BitShiftNumber=8  BitShiftDirection=Right
  Shift Arithmetic2 : ArithShift  BitShiftNumber=16  BitShiftDirection=Right
  Shift Arithmetic3 : ArithShift  BitShiftNumber=24  BitShiftDirection=Right
  Shift Arithmetic4 : ArithShift  BitShiftNumber=8  BitShiftDirection=Right
  MSG : Outport  OutDataTypeStr=uint16
  wires:
  Shift Arithmetic1/1 -> Data Type Conversion3/1
  Shift Arithmetic3/1 -> Data Type Conversion5/1
  Constant3/1 -> Shift Arithmetic3/1, Shift Arithmetic2/1, Shift Arithmetic1/1, Data Type Conversion2/1
  Mux3/1 -> Data Type Conversion/1
  Constant8/1 -> Mux3/1
  Data Type Conversion3/1 -> Mux3/6
  Data Type Conversion2/1 -> Mux3/5
  Data Type Conversion1/1 -> Mux3/3
  Data Type Conversion5/1 -> Mux3/8
  Current/1 -> Shift Arithmetic4/1, Data Type Conversion1/1
  Shift Arithmetic2/1 -> Data Type Conversion4/1
  Constant1/1 -> Mux3/2
  Data Type Conversion6/1 -> Mux3/4
  Shift Arithmetic4/1 -> Data Type Conversion6/1
  Data Type Conversion4/1 -> Mux3/7
  Data Type Conversion/1 -> MSG/1

== system ZeroForceDrag_SingleJoint/DynamicCalculation/DriveMotor/驱动器指令/Chart2/TF/J4_TF ==
  note: 电流
  note: 位
      | 置
  note: 命令
  Current : Inport
  Constant1 : Constant  Value=hex2dec('46')  OutDataTypeStr=uint8
  Constant3 : Constant  Value=0  VectorParams1D=off  OutDataTypeStr=uint8  SampleTime=-1
  Constant8 : Constant  Value=hex2dec('54')  OutDataTypeStr=uint8
  Data Type Conversion : DataTypeConversion  OutDataTypeStr=uint16
  Data Type Conversion{1..6} (6 alike) : DataTypeConversion  OutDataTypeStr=uint8
  Mux3 : Mux  Inputs=8
  Shift Arithmetic1 : ArithShift  BitShiftNumber=8  BitShiftDirection=Right
  Shift Arithmetic2 : ArithShift  BitShiftNumber=16  BitShiftDirection=Right
  Shift Arithmetic3 : ArithShift  BitShiftNumber=24  BitShiftDirection=Right
  Shift Arithmetic4 : ArithShift  BitShiftNumber=8  BitShiftDirection=Right
  MSG : Outport  OutDataTypeStr=uint16
  wires:
  Data Type Conversion/1 -> MSG/1
  Data Type Conversion4/1 -> Mux3/7
  Shift Arithmetic4/1 -> Data Type Conversion6/1
  Data Type Conversion6/1 -> Mux3/4
  Constant1/1 -> Mux3/2
  Shift Arithmetic2/1 -> Data Type Conversion4/1
  Current/1 -> Data Type Conversion1/1, Shift Arithmetic4/1
  Data Type Conversion5/1 -> Mux3/8
  Data Type Conversion1/1 -> Mux3/3
  Data Type Conversion2/1 -> Mux3/5
  Data Type Conversion3/1 -> Mux3/6
  Constant8/1 -> Mux3/1
  Mux3/1 -> Data Type Conversion/1
  Constant3/1 -> Data Type Conversion2/1, Shift Arithmetic1/1, Shift Arithmetic2/1, Shift Arithmetic3/1
  Shift Arithmetic3/1 -> Data Type Conversion5/1
  Shift Arithmetic1/1 -> Data Type Conversion3/1

== system ZeroForceDrag_SingleJoint/DynamicCalculation/DriveMotor/驱动器指令/Chart2/TF/J5_TF ==
  note: 命令
  note: 位
      | 置
  note: 电流
  Current : Inport
  Constant1 : Constant  Value=hex2dec('46')  OutDataTypeStr=uint8
  Constant3 : Constant  Value=0  VectorParams1D=off  OutDataTypeStr=uint8  SampleTime=-1
  Constant8 : Constant  Value=hex2dec('54')  OutDataTypeStr=uint8
  Data Type Conversion : DataTypeConversion  OutDataTypeStr=uint16
  Data Type Conversion{1..6} (6 alike) : DataTypeConversion  OutDataTypeStr=uint8
  Mux3 : Mux  Inputs=8
  Shift Arithmetic1 : ArithShift  BitShiftNumber=8  BitShiftDirection=Right
  Shift Arithmetic2 : ArithShift  BitShiftNumber=16  BitShiftDirection=Right
  Shift Arithmetic3 : ArithShift  BitShiftNumber=24  BitShiftDirection=Right
  Shift Arithmetic4 : ArithShift  BitShiftNumber=8  BitShiftDirection=Right
  MSG : Outport  OutDataTypeStr=uint16
  wires:
  Shift Arithmetic1/1 -> Data Type Conversion3/1
  Shift Arithmetic3/1 -> Data Type Conversion5/1
  Constant3/1 -> Shift Arithmetic3/1, Shift Arithmetic2/1, Shift Arithmetic1/1, Data Type Conversion2/1
  Mux3/1 -> Data Type Conversion/1
  Constant8/1 -> Mux3/1
  Data Type Conversion3/1 -> Mux3/6
  Data Type Conversion2/1 -> Mux3/5
  Data Type Conversion1/1 -> Mux3/3
  Data Type Conversion5/1 -> Mux3/8
  Current/1 -> Shift Arithmetic4/1, Data Type Conversion1/1
  Shift Arithmetic2/1 -> Data Type Conversion4/1
  Constant1/1 -> Mux3/2
  Data Type Conversion6/1 -> Mux3/4
  Shift Arithmetic4/1 -> Data Type Conversion6/1
  Data Type Conversion4/1 -> Mux3/7
  Data Type Conversion/1 -> MSG/1

== system ZeroForceDrag_SingleJoint/DynamicCalculation/DriveMotor/驱动器指令/Chart2/TF/J6_TF ==
  note: 电流
  note: 位
      | 置
  note: 命令
  Current : Inport
  Constant1 : Constant  Value=hex2dec('46')  OutDataTypeStr=uint8
  Constant3 : Constant  Value=0  VectorParams1D=off  OutDataTypeStr=uint8  SampleTime=-1
  Constant8 : Constant  Value=hex2dec('54')  OutDataTypeStr=uint8
  Data Type Conversion : DataTypeConversion  OutDataTypeStr=uint16
  Data Type Conversion{1..6} (6 alike) : DataTypeConversion  OutDataTypeStr=uint8
  Mux3 : Mux  Inputs=8
  Shift Arithmetic1 : ArithShift  BitShiftNumber=8  BitShiftDirection=Right
  Shift Arithmetic2 : ArithShift  BitShiftNumber=16  BitShiftDirection=Right
  Shift Arithmetic3 : ArithShift  BitShiftNumber=24  BitShiftDirection=Right
  Shift Arithmetic4 : ArithShift  BitShiftNumber=8  BitShiftDirection=Right
  MSG : Outport  OutDataTypeStr=uint16
  wires:
  Data Type Conversion/1 -> MSG/1
  Data Type Conversion4/1 -> Mux3/7
  Shift Arithmetic4/1 -> Data Type Conversion6/1
  Data Type Conversion6/1 -> Mux3/4
  Constant1/1 -> Mux3/2
  Shift Arithmetic2/1 -> Data Type Conversion4/1
  Current/1 -> Data Type Conversion1/1, Shift Arithmetic4/1
  Data Type Conversion5/1 -> Mux3/8
  Data Type Conversion1/1 -> Mux3/3
  Data Type Conversion2/1 -> Mux3/5
  Data Type Conversion3/1 -> Mux3/6
  Constant8/1 -> Mux3/1
  Mux3/1 -> Data Type Conversion/1
  Constant3/1 -> Data Type Conversion2/1, Shift Arithmetic1/1, Shift Arithmetic2/1, Shift Arithmetic3/1
  Shift Arithmetic3/1 -> Data Type Conversion5/1
  Shift Arithmetic1/1 -> Data Type Conversion3/1

== system ZeroForceDrag_SingleJoint/DynamicCalculation/DriveMotor/驱动器指令/Chart2/UM1/J1_UM1 ==
  note: 命令
  note: 位
      | 置
  note: 电流
  Constant1 : Constant  Value=hex2dec('4d')  OutDataTypeStr=uint8
  Constant2 : Constant  Value=0  VectorParams1D=off  OutDataTypeStr=uint8  SampleTime=-1
  Constant3 : Constant  VectorParams1D=off  OutDataTypeStr=uint8  SampleTime=-1
  Constant8 : Constant  Value=hex2dec('55')  OutDataTypeStr=uint8
  Data Type Conversion : DataTypeConversion  OutDataTypeStr=uint16
  Data Type Conversion{1..6} (6 alike) : DataTypeConversion  OutDataTypeStr=uint8
  Mux3 : Mux  Inputs=8
  Shift Arithmetic1 : ArithShift  BitShiftNumber=8  BitShiftDirection=Right
  Shift Arithmetic2 : ArithShift  BitShiftNumber=16  BitShiftDirection=Right
  Shift Arithmetic3 : ArithShift  BitShiftNumber=24  BitShiftDirection=Right
  Shift Arithmetic4 : ArithShift  BitShiftNumber=8  BitShiftDirection=Right
  MSG : Outport
  wires:
  Constant3/1 -> Shift Arithmetic3/1, Shift Arithmetic2/1, Data Type Conversion2/1, Shift Arithmetic1/1
  Data Type Conversion2/1 -> Mux3/5
  Data Type Conversion4/1 -> Mux3/7
  Mux3/1 -> Data Type Conversion/1
  Data Type Conversion6/1 -> Mux3/4
  Data Type Conversion/1 -> MSG/1
  Shift Arithmetic3/1 -> Data Type Conversion5/1
  Constant2/1 -> Data Type Conversion1/1, Shift Arithmetic4/1
  Data Type Conversion3/1 -> Mux3/6
  Constant8/1 -> Mux3/1
  Shift Arithmetic1/1 -> Data Type Conversion3/1
  Shift Arithmetic4/1 -> Data Type Conversion6/1
  Constant1/1 -> Mux3/2
  Data Type Conversion1/1 -> Mux3/3
  Shift Arithmetic2/1 -> Data Type Conversion4/1
  Data Type Conversion5/1 -> Mux3/8

== system ZeroForceDrag_SingleJoint/DynamicCalculation/DriveMotor/驱动器指令/Chart2/UM1/J2_UM1 ==
  note: 电流
  note: 位
      | 置
  note: 命令
  Constant1 : Constant  Value=hex2dec('4d')  OutDataTypeStr=uint8
  Constant2 : Constant  Value=0  VectorParams1D=off  OutDataTypeStr=uint8  SampleTime=-1
  Constant3 : Constant  VectorParams1D=off  OutDataTypeStr=uint8  SampleTime=-1
  Constant8 : Constant  Value=hex2dec('55')  OutDataTypeStr=uint8
  Data Type Conversion : DataTypeConversion  OutDataTypeStr=uint16
  Data Type Conversion{1..6} (6 alike) : DataTypeConversion  OutDataTypeStr=uint8
  Mux3 : Mux  Inputs=8
  Shift Arithmetic1 : ArithShift  BitShiftNumber=8  BitShiftDirection=Right
  Shift Arithmetic2 : ArithShift  BitShiftNumber=16  BitShiftDirection=Right
  Shift Arithmetic3 : ArithShift  BitShiftNumber=24  BitShiftDirection=Right
  Shift Arithmetic4 : ArithShift  BitShiftNumber=8  BitShiftDirection=Right
  MSG : Outport
  wires:
  Data Type Conversion5/1 -> Mux3/8
  Shift Arithmetic2/1 -> Data Type Conversion4/1
  Data Type Conversion1/1 -> Mux3/3
  Constant1/1 -> Mux3/2
  Shift Arithmetic4/1 -> Data Type Conversion6/1
  Shift Arithmetic1/1 -> Data Type Conversion3/1
  Constant8/1 -> Mux3/1
  Data Type Conversion3/1 -> Mux3/6
  Constant2/1 -> Shift Arithmetic4/1, Data Type Conversion1/1
  Shift Arithmetic3/1 -> Data Type Conversion5/1
  Data Type Conversion/1 -> MSG/1
  Data Type Conversion6/1 -> Mux3/4
  Mux3/1 -> Data Type Conversion/1
  Data Type Conversion4/1 -> Mux3/7
  Data Type Conversion2/1 -> Mux3/5
  Constant3/1 -> Shift Arithmetic1/1, Data Type Conversion2/1, Shift Arithmetic2/1, Shift Arithmetic3/1

== system ZeroForceDrag_SingleJoint/DynamicCalculation/DriveMotor/驱动器指令/Chart2/UM1/J3_UM1 ==
  note: 命令
  note: 位
      | 置
  note: 电流
  Constant1 : Constant  Value=hex2dec('4d')  OutDataTypeStr=uint8
  Constant2 : Constant  Value=0  VectorParams1D=off  OutDataTypeStr=uint8  SampleTime=-1
  Constant3 : Constant  VectorParams1D=off  OutDataTypeStr=uint8  SampleTime=-1
  Constant8 : Constant  Value=hex2dec('55')  OutDataTypeStr=uint8
  Data Type Conversion : DataTypeConversion  OutDataTypeStr=uint16
  Data Type Conversion{1..6} (6 alike) : DataTypeConversion  OutDataTypeStr=uint8
  Mux3 : Mux  Inputs=8
  Shift Arithmetic1 : ArithShift  BitShiftNumber=8  BitShiftDirection=Right
  Shift Arithmetic2 : ArithShift  BitShiftNumber=16  BitShiftDirection=Right
  Shift Arithmetic3 : ArithShift  BitShiftNumber=24  BitShiftDirection=Right
  Shift Arithmetic4 : ArithShift  BitShiftNumber=8  BitShiftDirection=Right
  MSG : Outport
  wires:
  Constant3/1 -> Shift Arithmetic3/1, Shift Arithmetic2/1, Data Type Conversion2/1, Shift Arithmetic1/1
  Data Type Conversion2/1 -> Mux3/5
  Data Type Conversion4/1 -> Mux3/7
  Mux3/1 -> Data Type Conversion/1
  Data Type Conversion6/1 -> Mux3/4
  Data Type Conversion/1 -> MSG/1
  Shift Arithmetic3/1 -> Data Type Conversion5/1
  Constant2/1 -> Data Type Conversion1/1, Shift Arithmetic4/1
  Data Type Conversion3/1 -> Mux3/6
  Constant8/1 -> Mux3/1
  Shift Arithmetic1/1 -> Data Type Conversion3/1
  Shift Arithmetic4/1 -> Data Type Conversion6/1
  Constant1/1 -> Mux3/2
  Data Type Conversion1/1 -> Mux3/3
  Shift Arithmetic2/1 -> Data Type Conversion4/1
  Data Type Conversion5/1 -> Mux3/8

== system ZeroForceDrag_SingleJoint/DynamicCalculation/DriveMotor/驱动器指令/Chart2/UM1/J4_UM1 ==
  note: 电流
  note: 位
      | 置
  note: 命令
  Constant1 : Constant  Value=hex2dec('4d')  OutDataTypeStr=uint8
  Constant2 : Constant  Value=0  VectorParams1D=off  OutDataTypeStr=uint8  SampleTime=-1
  Constant3 : Constant  VectorParams1D=off  OutDataTypeStr=uint8  SampleTime=-1
  Constant8 : Constant  Value=hex2dec('55')  OutDataTypeStr=uint8
  Data Type Conversion : DataTypeConversion  OutDataTypeStr=uint16
  Data Type Conversion{1..6} (6 alike) : DataTypeConversion  OutDataTypeStr=uint8
  Mux3 : Mux  Inputs=8
  Shift Arithmetic1 : ArithShift  BitShiftNumber=8  BitShiftDirection=Right
  Shift Arithmetic2 : ArithShift  BitShiftNumber=16  BitShiftDirection=Right
  Shift Arithmetic3 : ArithShift  BitShiftNumber=24  BitShiftDirection=Right
  Shift Arithmetic4 : ArithShift  BitShiftNumber=8  BitShiftDirection=Right
  MSG : Outport
  wires:
  Data Type Conversion5/1 -> Mux3/8
  Shift Arithmetic2/1 -> Data Type Conversion4/1
  Data Type Conversion1/1 -> Mux3/3
  Constant1/1 -> Mux3/2
  Shift Arithmetic4/1 -> Data Type Conversion6/1
  Shift Arithmetic1/1 -> Data Type Conversion3/1
  Constant8/1 -> Mux3/1
  Data Type Conversion3/1 -> Mux3/6
  Constant2/1 -> Shift Arithmetic4/1, Data Type Conversion1/1
  Shift Arithmetic3/1 -> Data Type Conversion5/1
  Data Type Conversion/1 -> MSG/1
  Data Type Conversion6/1 -> Mux3/4
  Mux3/1 -> Data Type Conversion/1
  Data Type Conversion4/1 -> Mux3/7
  Data Type Conversion2/1 -> Mux3/5
  Constant3/1 -> Shift Arithmetic1/1, Data Type Conversion2/1, Shift Arithmetic2/1, Shift Arithmetic3/1

== system ZeroForceDrag_SingleJoint/DynamicCalculation/DriveMotor/驱动器指令/Chart2/UM1/J5_UM1 ==
  note: 命令
  note: 位
      | 置
  note: 电流
  Constant1 : Constant  Value=hex2dec('4d')  OutDataTypeStr=uint8
  Constant2 : Constant  Value=0  VectorParams1D=off  OutDataTypeStr=uint8  SampleTime=-1
  Constant3 : Constant  VectorParams1D=off  OutDataTypeStr=uint8  SampleTime=-1
  Constant8 : Constant  Value=hex2dec('55')  OutDataTypeStr=uint8
  Data Type Conversion : DataTypeConversion  OutDataTypeStr=uint16
  Data Type Conversion{1..6} (6 alike) : DataTypeConversion  OutDataTypeStr=uint8
  Mux3 : Mux  Inputs=8
  Shift Arithmetic1 : ArithShift  BitShiftNumber=8  BitShiftDirection=Right
  Shift Arithmetic2 : ArithShift  BitShiftNumber=16  BitShiftDirection=Right
  Shift Arithmetic3 : ArithShift  BitShiftNumber=24  BitShiftDirection=Right
  Shift Arithmetic4 : ArithShift  BitShiftNumber=8  BitShiftDirection=Right
  MSG : Outport
  wires:
  Constant3/1 -> Shift Arithmetic3/1, Shift Arithmetic2/1, Data Type Conversion2/1, Shift Arithmetic1/1
  Data Type Conversion2/1 -> Mux3/5
  Data Type Conversion4/1 -> Mux3/7
  Mux3/1 -> Data Type Conversion/1
  Data Type Conversion6/1 -> Mux3/4
  Data Type Conversion/1 -> MSG/1
  Shift Arithmetic3/1 -> Data Type Conversion5/1
  Constant2/1 -> Data Type Conversion1/1, Shift Arithmetic4/1
  Data Type Conversion3/1 -> Mux3/6
  Constant8/1 -> Mux3/1
  Shift Arithmetic1/1 -> Data Type Conversion3/1
  Shift Arithmetic4/1 -> Data Type Conversion6/1
  Constant1/1 -> Mux3/2
  Data Type Conversion1/1 -> Mux3/3
  Shift Arithmetic2/1 -> Data Type Conversion4/1
  Data Type Conversion5/1 -> Mux3/8

== system ZeroForceDrag_SingleJoint/DynamicCalculation/DriveMotor/驱动器指令/Chart2/UM1/J6_UM1 ==
  note: 电流
  note: 位
      | 置
  note: 命令
  Constant1 : Constant  Value=hex2dec('4d')  OutDataTypeStr=uint8
  Constant2 : Constant  Value=0  VectorParams1D=off  OutDataTypeStr=uint8  SampleTime=-1
  Constant3 : Constant  VectorParams1D=off  OutDataTypeStr=uint8  SampleTime=-1
  Constant8 : Constant  Value=hex2dec('55')  OutDataTypeStr=uint8
  Data Type Conversion : DataTypeConversion  OutDataTypeStr=uint16
  Data Type Conversion{1..6} (6 alike) : DataTypeConversion  OutDataTypeStr=uint8
  Mux3 : Mux  Inputs=8
  Shift Arithmetic1 : ArithShift  BitShiftNumber=8  BitShiftDirection=Right
  Shift Arithmetic2 : ArithShift  BitShiftNumber=16  BitShiftDirection=Right
  Shift Arithmetic3 : ArithShift  BitShiftNumber=24  BitShiftDirection=Right
  Shift Arithmetic4 : ArithShift  BitShiftNumber=8  BitShiftDirection=Right
  MSG : Outport
  wires:
  Data Type Conversion5/1 -> Mux3/8
  Shift Arithmetic2/1 -> Data Type Conversion4/1
  Data Type Conversion1/1 -> Mux3/3
  Constant1/1 -> Mux3/2
  Shift Arithmetic4/1 -> Data Type Conversion6/1
  Shift Arithmetic1/1 -> Data Type Conversion3/1
  Constant8/1 -> Mux3/1
  Data Type Conversion3/1 -> Mux3/6
  Constant2/1 -> Shift Arithmetic4/1, Data Type Conversion1/1
  Shift Arithmetic3/1 -> Data Type Conversion5/1
  Data Type Conversion/1 -> MSG/1
  Data Type Conversion6/1 -> Mux3/4
  Mux3/1 -> Data Type Conversion/1
  Data Type Conversion4/1 -> Mux3/7
  Data Type Conversion2/1 -> Mux3/5
  Constant3/1 -> Shift Arithmetic1/1, Data Type Conversion2/1, Shift Arithmetic2/1, Shift Arithmetic3/1
